simulink model "Control2"  (Simulink 9.0)
settings: Solver=VariableStepAuto  StartTime=0.0  StopTime=2  EnableMultiTasking=on
values from neighbouring files (symbols this model uses):
  Kd = Kp*tau    [Control_Disc.m]    (also in Control_PID.m; Controladores.m; PD_Feedforward.m; dsgn_PD.m = Kp.*Td)
  Ki = [0 0 0]    [Control_Disc.m]    (also in Control_PID.m = [0 0 0]'; Controladores.m; PD_Feedforward.m; dsgn_PD.m = Kp./Ti)
  Kp = [7.4989e+04 1.4125e+05 1.5488e+04]    [Control_Disc.m]    (also in Control_PID.m = [7.4989e+04 1.4125e+05 1.5488e+04]'; Controladores.m; PD_Feedforward.m; dsgn_PD.m = [2.1312e+06 8.4844e+05 4.5042e+05])
undefined symbols (not defined in the file or in its folder): CinematicaDirecta
settings Model: Creator=Manuel G. Ortega  LastModifiedBy=Raúl  ExtModeTrigMode=oneshot  ExtModeArmWhenConnect=off
settings SolverCC: AlgebraicLoopSolver=LineSearch
settings DataIOCC: SignalLoggingSaveFormat=ModelDataLogs
settings OptimizationCC: BooleanDataType=off  ExpressionDepthLimit=2147483647  InitFltsAndDblsToZero=on
settings DebuggingCC: SaveWithParameterizedLinksMsg=none  SignalResolutionControl=TryResolveAllWithWarning  MultiTaskDSMMsg=warning  MultiTaskCondExecSysMsg=none  FcnCallInpInsideContextMsg=warning  StateNameClashWarn=warning  StrictBusMsg=None
settings HardwareCC: TargetUnknown=on
settings GRTTargetCC: TargetFcnLib=ansi_tfl_tmw.mat  GeneratePreprocessorConditionals=Disable all  CombineOutputUpdateFcns=off  GRTInterface=on
settings ConfigComp: CovSFcnEnable=off

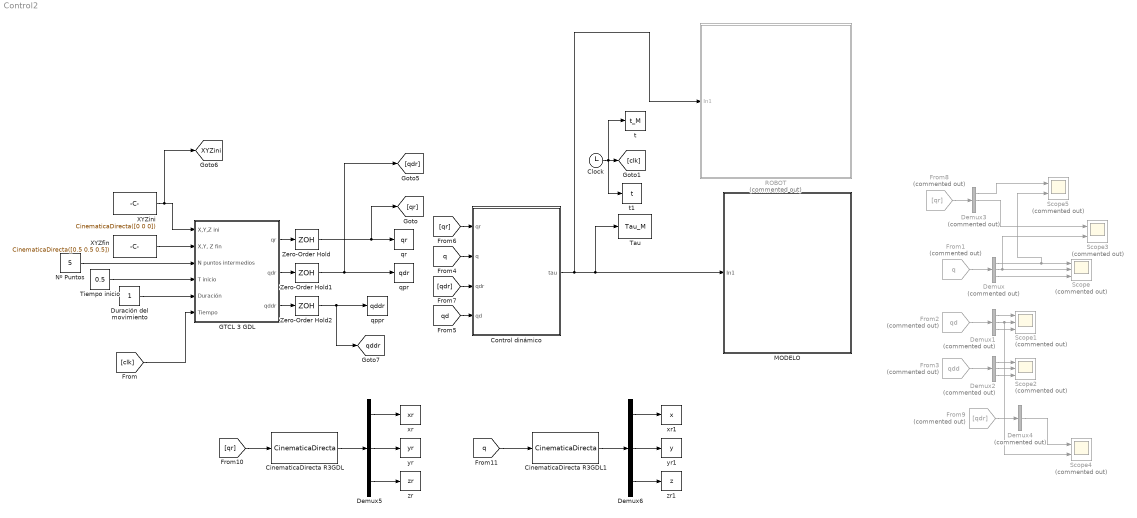
== system Control2 ==
  CinematicaDirecta R3GDL : MATLABFcn  MATLABFcn=CinematicaDirecta
  CinematicaDirecta R3GDL1 : MATLABFcn  MATLABFcn=CinematicaDirecta
  Clock : Clock
  "Control dinámico " : Subsystem
  Demux{,1..4} (5 alike) : Demux  Commented=on  Outputs=3
  Demux5 : Demux  Outputs=3
  Demux6 : Demux  Outputs=3
  Duración del movimiento : Constant
  From1 : From  Commented=on  GotoTag=q
  From2 : From  Commented=on  GotoTag=qd
  From3 : From  Commented=on  GotoTag=qdd
  From8 : From  Commented=on  GotoTag=qr
  From9 : From  Commented=on  GotoTag=qdr
  GTCL 3 GDL : Subsystem
  MODELO : Subsystem
  Nº Puntos : Constant  Value=5
  "ROBOT " : Subsystem  Commented=on
  Scope : Scope  Commented=on  NumInputPorts=3
  Scope1 : Scope  Commented=on  NumInputPorts=3
  Scope2 : Scope  Commented=on  NumInputPorts=3
  Scope3 : Scope  Commented=on  NumInputPorts=2
  Scope4 : Scope  Commented=on  NumInputPorts=2
  Scope5 : Scope  Commented=on  NumInputPorts=2
  "Tau " : ToWorkspace  VariableName=Tau_M  SampleTime=-1
  Tiempo inicio : Constant  Value=0.5
  XYZfin : Constant  Value=CinematicaDirecta([0.5 0.5 0.5])
  XYZini : Constant  Value=CinematicaDirecta([0 0 0])
  Zero-Order Hold : ZeroOrderHold  SampleTime=15e-3
  Zero-Order Hold1 : ZeroOrderHold  SampleTime=15e-3
  Zero-Order Hold2 : ZeroOrderHold  SampleTime=15e-3
  qppr : ToWorkspace  VariableName=qddr
  qpr : ToWorkspace  VariableName=qdr
  qr : ToWorkspace  VariableName=qr
  t : ToWorkspace  VariableName=t_M  SampleTime=-1
  t1 : ToWorkspace  VariableName=t  SampleTime=-1
  xr : ToWorkspace  VariableName=xr  SampleTime=-1
  xr1 : ToWorkspace  VariableName=x  SampleTime=-1
  yr : ToWorkspace  VariableName=yr  SampleTime=-1
  yr1 : ToWorkspace  VariableName=y  SampleTime=-1
  zr : ToWorkspace  VariableName=zr  SampleTime=-1
  zr1 : ToWorkspace  VariableName=z  SampleTime=-1
  tag scope: XYZini=global, qddr=global
  wires:
  "Control dinámico "/1(tau) -> "ROBOT "/1(In1), MODELO/1(In1), "Tau "/1
  Demux/1 -> Scope5/2, Scope/1
  Demux/2 -> Scope3/2, Scope/2
  Demux/3 -> Scope/3
  Demux1/3 -> Scope1/3
  Demux1/1 -> Scope1/1
  Demux2/1 -> Scope2/1
  Demux2/2 -> Scope2/2
  Demux2/3 -> Scope2/3
  XYZini/1 -> [XYZini], GTCL 3 GDL/1(X,Y,Z ini)
  XYZfin/1 -> GTCL 3 GDL/2("X,Y, Z fin")
  Nº Puntos/1 -> GTCL 3 GDL/3(N puntos intermedios)
  Tiempo inicio/1 -> GTCL 3 GDL/4(T inicio)
  Duración del movimiento/1 -> GTCL 3 GDL/5(Duración)
  [clk] -> GTCL 3 GDL/6(Tiempo)
  Clock/1 -> t1/1, t/1, [clk]
  From1/1 -> Demux/1
  From3/1 -> Demux2/1
  From2/1 -> Demux1/1
  [qr] -> "Control dinámico "/1(qr)
  [qdr] -> "Control dinámico "/3(qdr)
  [qd] -> "Control dinámico "/4(qd)
  [q] -> "Control dinámico "/2(q)
  From8/1 -> Demux3/1
  Demux3/2 -> Scope3/1
  Demux4/2 -> Scope4/1
  From9/1 -> Demux4/1
  Demux1/2 -> Scope4/2, Scope1/2
  Demux3/1 -> Scope5/1
  CinematicaDirecta R3GDL/1 -> Demux5/1
  [qr] -> CinematicaDirecta R3GDL/1
  Demux5/2 -> yr/1
  Demux5/1 -> xr/1
  Demux5/3 -> zr/1
  Demux6/3 -> zr1/1
  Demux6/1 -> xr1/1
  Demux6/2 -> yr1/1
  [q] -> CinematicaDirecta R3GDL1/1
  CinematicaDirecta R3GDL1/1 -> Demux6/1
  GTCL 3 GDL/1(qr) -> Zero-Order Hold/1
  GTCL 3 GDL/2(qdr) -> Zero-Order Hold1/1
  GTCL 3 GDL/3(qddr) -> Zero-Order Hold2/1
  Zero-Order Hold2/1 -> [qddr], qppr/1
  Zero-Order Hold1/1 -> [qdr], qpr/1
  Zero-Order Hold/1 -> [qr], qr/1

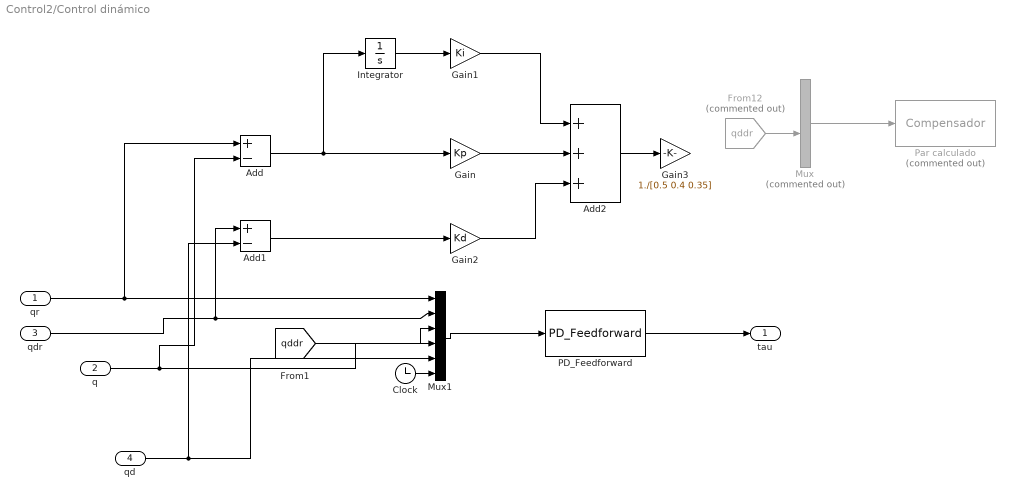
== system Control2/Control dinámico  ==
  qr : Inport
  q : Inport  Port=2
  qdr : Inport  Port=3
  qd : Inport  Port=4
  Add : Sum  Inputs=+-
  Add1 : Sum  Inputs=+-
  Add2 : Sum  Inputs=+++
  Clock : Clock
  From12 : From  Commented=on  GotoTag=qddr  TagVisibility=global
  Gain : Gain  Gain=Kp
  Gain1 : Gain  Gain=Ki
  Gain2 : Gain  Gain=Kd
  Gain3 : Gain  Gain=1./[0.5 0.4 0.35]
  Integrator : Integrator
  Mux : Mux  Commented=on
  Mux1 : Mux  Inputs=6
  "PD_Feedforward " : MATLABFcn  MATLABFcn=PD_Feedforward  SampleTime=1e-3
  "Par calculado " : MATLABFcn  Commented=on  MATLABFcn=Compensador
  tau : Outport
  wires:
  Add/1 -> Integrator/1, Gain/1
  Add1/1 -> Gain2/1
  Integrator/1 -> Gain1/1
  Gain1/1 -> Add2/1
  Gain/1 -> Add2/2
  Gain2/1 -> Add2/3
  Mux/1 -> "Par calculado "/1
  From12/1 -> Mux/3
  Mux1/1 -> "PD_Feedforward "/1
  qr/1 -> Add/1, Mux1/1
  qdr/1 -> Add1/1, Mux1/2
  [qddr] -> Mux1/3
  q/1 -> Add/2, Mux1/4
  qd/1 -> Add1/2, Mux1/5
  Add2/1 -> Gain3/1
  "PD_Feedforward "/1 -> tau/1
  Clock/1 -> Mux1/6

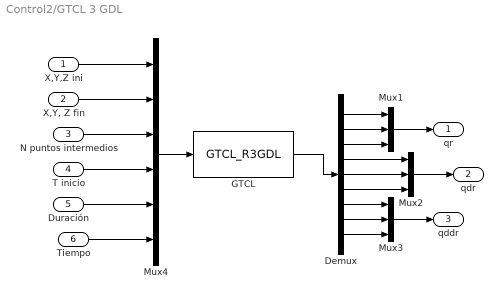
== system Control2/GTCL 3 GDL ==
  X,Y,Z ini : Inport
  "X,Y, Z fin" : Inport  Port=2
  N puntos intermedios : Inport  Port=3
  T inicio : Inport  Port=4
  Duración : Inport  Port=5
  Tiempo : Inport  Port=6
  Demux : Demux  Outputs=9
  GTCL : MATLABFcn  MATLABFcn=GTCL_R3GDL  OutputDimensions=9
  Mux1 : Mux  Inputs=3
  Mux2 : Mux  Inputs=3
  Mux3 : Mux  Inputs=3
  Mux4 : Mux  Inputs=6
  qr : Outport
  qdr : Outport  Port=2
  qddr : Outport  Port=3
  wires:
  Demux/9 -> Mux3/3
  Demux/8 -> Mux3/2
  Demux/7 -> Mux3/1
  Mux3/1 -> qddr/1
  Demux/6 -> Mux2/3
  Demux/5 -> Mux2/2
  Demux/4 -> Mux2/1
  Mux2/1 -> qdr/1
  Demux/3 -> Mux1/3
  Demux/2 -> Mux1/2
  Demux/1 -> Mux1/1
  GTCL/1 -> Demux/1
  Tiempo/1 -> Mux4/6
  Duración/1 -> Mux4/5
  T inicio/1 -> Mux4/4
  N puntos intermedios/1 -> Mux4/3
  "X,Y, Z fin"/1 -> Mux4/2
  X,Y,Z ini/1 -> Mux4/1
  Mux4/1 -> GTCL/1
  Mux1/1 -> qr/1

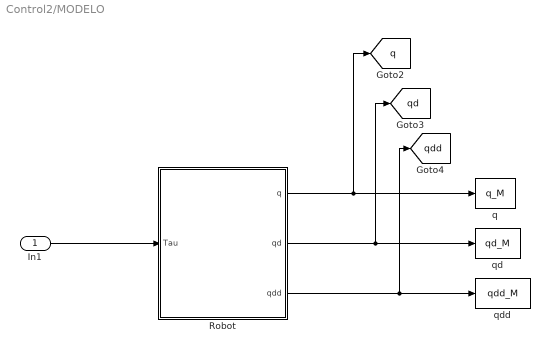
== system Control2/MODELO ==
  In1 : Inport
  Robot : Subsystem
  q : ToWorkspace  VariableName=q_M  SampleTime=-1
  qd : ToWorkspace  VariableName=qd_M  SampleTime=-1
  qdd : ToWorkspace  VariableName=qdd_M  SampleTime=-1
  tag scope: q=global, qd=global, qdd=global
  wires:
  Robot/2(qd) -> [qd], qd/1
  Robot/3(qdd) -> [qdd], qdd/1
  Robot/1(q) -> [q], q/1
  In1/1 -> Robot/1(Tau)

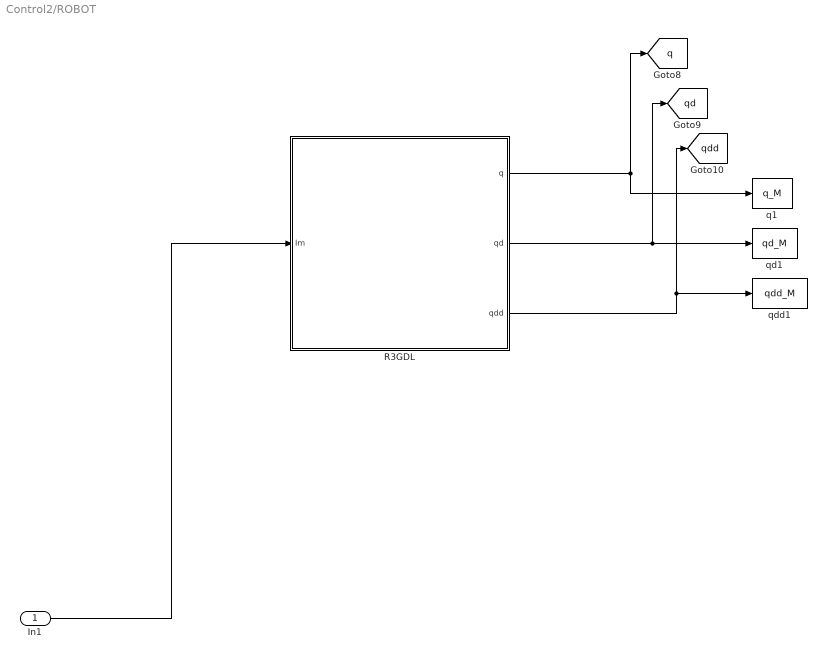
== system Control2/ROBOT  ==
  In1 : Inport
  R3GDL : Subsystem  mask(Control y Programación de Robots (4 GIERM)){NGrupo=3, q1_ini=0, q2_ini=0, q3_ini=0, Bl_q1=off, Bl_q2=off, Bl_q3=off, AccionamientoDirecto=on}
      mask prompts: NGrupo "Nº de GRUPO"; q1_ini "q1 inicial  (rad)"; q2_ini "q2 inicial (rad)"; q3_ini "q3_inicial (rad)"; Bl_q1 "Bloqueo q1"; Bl_q2 "Bloqueo q2"; Bl_q3 "Bloqueo q3"; AccionamientoDirecto "Accionamiento directo"
      mask help: Robot de 3 grados de libertad RRR
      mask Display:
      | image(imread('R3GDL_RRR.JPG'));
      | port_label('output', 1, 'q');
      | port_label('output', 2, 'qd');
      | port_label('output', 3, 'qdd');
      | port_label('input', 1, 'Im')
  q1 : ToWorkspace  VariableName=q_M  SampleTime=-1
  qd1 : ToWorkspace  VariableName=qd_M  SampleTime=-1
  qdd1 : ToWorkspace  VariableName=qdd_M  SampleTime=-1
  tag scope: q=global, qd=global, qdd=global
  wires:
  R3GDL/3(qdd) -> [qdd], qdd1/1
  R3GDL/2(qd) -> [qd], qd1/1
  R3GDL/1(q) -> q1/1, [q]
  In1/1 -> R3GDL/1(Im)

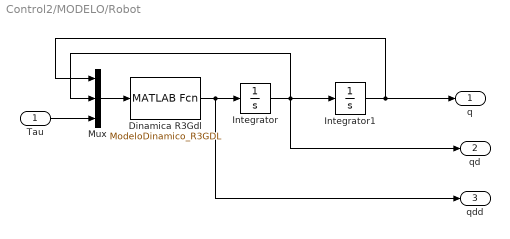
== system Control2/MODELO/Robot ==
  Tau : Inport
  Dinamica R3Gdl : MATLABFcn  MATLABFcn=ModeloDinamico_R3GDL
  Integrator : Integrator  InitialCondition=[0;0;0];
  Integrator1 : Integrator  InitialCondition=[0 0 0]
  Mux : Mux  Inputs=3
  q : Outport
  qd : Outport  Port=2
  qdd : Outport  Port=3
  wires:
  Mux/1 -> Dinamica R3Gdl/1
  Dinamica R3Gdl/1 -> Integrator/1, qdd/1
  Integrator/1 -> Mux/2, Integrator1/1, qd/1
  Integrator1/1 -> q/1, Mux/1
  Tau/1 -> Mux/3

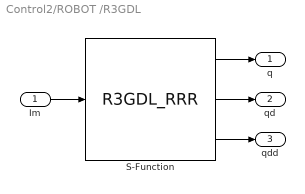
== system Control2/ROBOT /R3GDL ==
  Im : Inport
  S-Function : S-Function  FunctionName=R3GDL_RRR  Parameters=[q1_ini; q2_ini; q3_ini]; [Bl_q1; Bl_q2; Bl_q3]; AccionamientoDirecto; NGrupo  SFunctionDeploymentMode=off  EnableBusSupport=off
  q : Outport
  qd : Outport  Port=2
  qdd : Outport  Port=3
  wires:
  S-Function/3 -> qdd/1
  S-Function/2 -> qd/1
  S-Function/1 -> q/1
  Im/1 -> S-Function/1
